simulink model "RobotX_ss_acoustics_1019_bbox"  (R2014a)
settings: Solver=FixedStepDiscrete  StartTime=0.0  StopTime=inf  FixedStep=.25  RelTol=1e-3
undefined symbols (not defined in the file): Com1, Com2, Com3, Com4, DiscIntNeverNeededParam, standard
libraries: xpcseriallib x14, dspmtrx3 x3, slrtlib x3, simulink x2, speedgoatlib x1, speedgoatlib_IO102 x1
(part 2 of 3)

== matlab function RobotX_ss_acoustics_1019_bbox/Main FSM/Start//Speedgate/entrance/GPSMove ==
  data: GoalNED input; X input; Finished output; valid output; Y input; Psi input; pts output
function [Finished,valid,pts] = GPSmove(GoalNED,X,Y,Psi)
%Written by Dylan DeGaetano on September 1, 2014
%Last edited by: Anderson Lebbad
%
%This function will go to a given NED cooridnate, last edit changed the
%goal pt and variable names

persistent Sample
if isempty(Sample)
Sample = 0;
end
Finished = 0;
pts = zeros(8,2);
%$Distance to object in meters
if Sample == 100
    Sample = 0;
end

if Sample == 0
    pts(1,1) = X+5*cos(Psi*pi/180);
    pts(1,2) = Y+5*cos(Psi*pi/180);
    pts(8,1) = GoalNED(1,1);
    pts(8,2) = GoalNED(1,2);
    pts(2,:) = pts(1,:) +(1*(GoalNED-pts(1,:))/7);
    pts(3,:) = pts(1,:) +(2*(GoalNED-pts(1,:))/7);
    pts(4,:) = pts(1,:) +(3*(GoalNED-pts(1,:))/7);
    pts(5,:) = pts(1,:) +(4*(GoalNED-pts(1,:))/7);
    pts(6,:) = pts(1,:) +(5*(GoalNED-pts(1,:))/7);
    pts(7,:) = pts(1,:) +(6*(GoalNED-pts(1,:))/7);
    Sample = 1; 
    valid = 1;
    
else 
    range = sqrt(sum((GoalNED - [X Y]).^2));
    if range <= 8
        Finished = 1;
    end
    valid = 0;
    Sample = Sample + 1;
end

== matlab function RobotX_ss_acoustics_1019_bbox/Main FSM/Start//Speedgate/exit/CalcTimes ==
  data: pts input; u input; Data output
function Data = calcTimes(pts, u)
%Written by Anderson Lebbad on August 9, 2014
%Last Edited: Dylan DeGaetano September 1, 2014

%Calculates times for the boat to get to points for a trajectory, and
%formats Data for communication

%Initialize
Data = zeros(24,1);
traj = zeros(8,3);
traj(:,1:2) = pts;



for k = 2:8
    %Calculate distance to travel from last point
    distTravel = sqrt(sum((pts(k-1,:)-pts(k,:)).^2));
    %Assume 1m per second speed
    traj(k,3) = traj(k-1,3) + distTravel;
    %Add time based off initial velocity to get to first point past initial
    if k == 2
        traj(k,3) = traj(k,3) + 2.5*abs(2-u);
    end
end


%Output Data
for i=1:8
    for j = 1:3
        Data(3*(i-1)+j) = traj(i,j);
    end
end

== matlab function RobotX_ss_acoustics_1019_bbox/Main FSM/Start//Speedgate/exit/GPSMove ==
  data: GoalNED input; X input; Finished output; valid output; Y input; Psi input; pts output
function [Finished,valid,pts] = GPSmove(GoalNED,X,Y,Psi)
%Written by Dylan DeGaetano on September 1, 2014
%Last edited by: Anderson Lebbad
%
%This function will go to a given NED cooridnate, last edit changed the
%goal pt and variable names

persistent Sample
if isempty(Sample)
Sample = 0;
end
Finished = 0;
pts = zeros(8,2);
%$Distance to object in meters
if Sample == 100
    Sample = 0;
end

if Sample == 0
    pts(1,1) = X+5*cos(Psi*pi/180);
    pts(1,2) = Y+5*cos(Psi*pi/180);
    pts(8,1) = GoalNED(1,1);
    pts(8,2) = GoalNED(1,2);
    pts(2,:) = pts(1,:) +(1*(GoalNED-pts(1,:))/7);
    pts(3,:) = pts(1,:) +(2*(GoalNED-pts(1,:))/7);
    pts(4,:) = pts(1,:) +(3*(GoalNED-pts(1,:))/7);
    pts(5,:) = pts(1,:) +(4*(GoalNED-pts(1,:))/7);
    pts(6,:) = pts(1,:) +(5*(GoalNED-pts(1,:))/7);
    pts(7,:) = pts(1,:) +(6*(GoalNED-pts(1,:))/7);
    Sample = 1; 
    valid = 1;
    
else 
    range = sqrt(sum((GoalNED - [X Y]).^2));
    if range <= 8
        Finished = 1;
    end
    valid = 0;
    Sample = Sample + 1;
end

== matlab function RobotX_ss_acoustics_1019_bbox/Main FSM/Termination/CalcTimes ==
  data: pts input; u input; Data output
function Data = calcTimes(pts, u)
%Written by Anderson Lebbad on August 9, 2014
%Last Edited: Dylan DeGaetano September 1, 2014

%Calculates times for the boat to get to points for a trajectory, and
%formats Data for communication

%Initialize
Data = zeros(24,1);
traj = zeros(8,3);
traj(:,1:2) = pts;



for k = 2:8
    %Calculate distance to travel from last point
    distTravel = sqrt(sum((pts(k-1,:)-pts(k,:)).^2));
    %Assume 1m per second speed
    traj(k,3) = traj(k-1,3) + distTravel;
    %Add time based off initial velocity to get to first point past initial
    if k == 2
        traj(k,3) = traj(k,3) + 2.5*abs(2-u);
    end
end


%Output Data
for i=1:8
    for j = 1:3
        Data(3*(i-1)+j) = traj(i,j);
    end
end

== matlab function RobotX_ss_acoustics_1019_bbox/Main FSM/Termination/GPSMove ==
  data: GoalNED input; X input; valid output; Y input; Psi input; pts output
function [valid,pts] = GPSmove(GoalNED,X,Y,Psi)
%Written by Dylan DeGaetano on September 1, 2014
%Last edited by: Anderson Lebbad
%
%This function will go to a given NED cooridnate, last edit changed the
%goal pt and variable names

persistent Sample
if isempty(Sample)
Sample = 0;
end

pts = zeros(8,2);
%$Distance to object in meters

if Sample == 0
    pts(1,1) = X+5*cos(Psi*pi/180);
    pts(1,2) = Y+5*cos(Psi*pi/180);
    pts(8,1) = GoalNED(1,1);
    pts(8,2) = GoalNED(1,2);
    pts(2,:) = pts(1,:) +(1*(GoalNED-pts(1,:))/7);
    pts(3,:) = pts(1,:) +(2*(GoalNED-pts(1,:))/7);
    pts(4,:) = pts(1,:) +(3*(GoalNED-pts(1,:))/7);
    pts(5,:) = pts(1,:) +(4*(GoalNED-pts(1,:))/7);
    pts(6,:) = pts(1,:) +(5*(GoalNED-pts(1,:))/7);
    pts(7,:) = pts(1,:) +(6*(GoalNED-pts(1,:))/7);
    Sample = 1; 
    valid = 1;
    
else
    valid = 0;
end

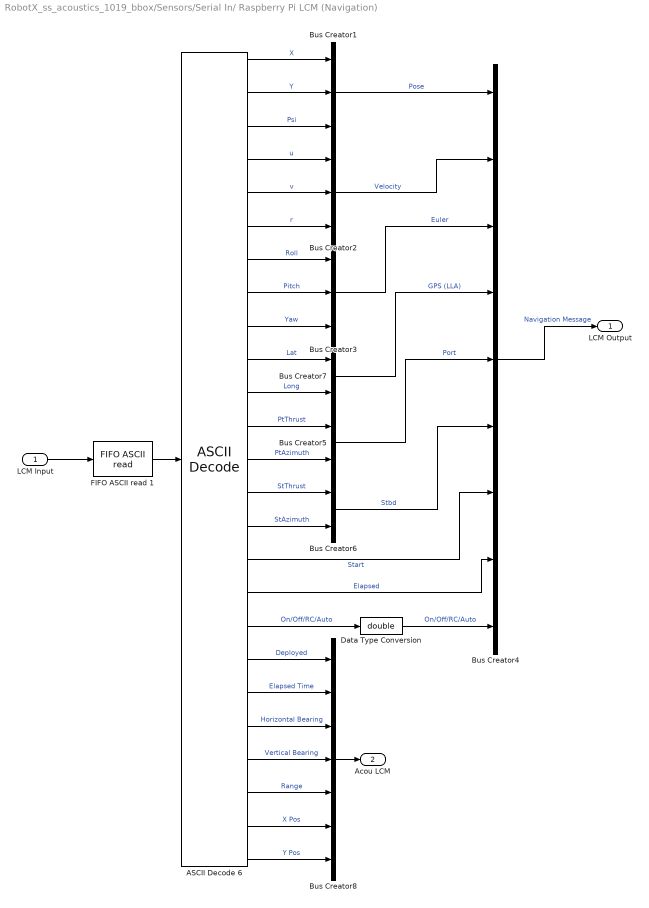
== system RobotX_ss_acoustics_1019_bbox/Sensors/Serial In/ Raspberry Pi LCM (Navigation) ==
  LCM Input : Inport
  ASCII Decode 6 : xpcseriallib/ASCII Decode   format=P1:%f P2:%f P3:%f V1:%f V2:%f V3:%f E1:%f E2:%f E3:%f Lat:%f Long:%f Pt1:%f Pt2:%f St1:%f St2:%f Start:%f Elapsed:%f RC:%d Deploy:%u Elapsed:%f Bearing1:%f Bearing2:%f Range:%f X_Pos:%f Y_Pos:%f \r\n  nvars=25  vartypes={}
  Bus Creator1 : BusCreator  Inputs=3
  Bus Creator2 : BusCreator  Inputs=3
  Bus Creator3 : BusCreator  Inputs=3
  Bus Creator4 : BusCreator  Inputs=9
  Bus Creator5 : BusCreator  Inputs=2
  Bus Creator6 : BusCreator  Inputs=2
  Bus Creator7 : BusCreator  Inputs=2
  Bus Creator8 : BusCreator  Inputs=7
  Data Type Conversion : DataTypeConversion  OutDataTypeStr=double
  FIFO ASCII read 1 : xpcseriallib/FIFO ASCII read   header={'P1:'}  term=[13 10]  hold=Zero output if no new data  enable=off  maxsize=1024  outputtype=8 bit uint null terminated  sampletime=-1
  LCM Output : Outport
  Acou LCM : Outport  Port=2
  wires:
  LCM Input/1 -> FIFO ASCII read 1/1
  FIFO ASCII read 1/1 -> ASCII Decode 6/1
  Bus Creator4/1 -> LCM Output/1  "Navigation Message"
  ASCII Decode 6/1 -> Bus Creator1/1  "X"
  ASCII Decode 6/2 -> Bus Creator1/2  "Y"
  ASCII Decode 6/3 -> Bus Creator1/3  "Psi"
  Bus Creator1/1 -> Bus Creator4/1  "Pose"
  ASCII Decode 6/4 -> Bus Creator2/1  "u"
  ASCII Decode 6/5 -> Bus Creator2/2  "v"
  Bus Creator2/1 -> Bus Creator4/2  "Velocity"
  ASCII Decode 6/7 -> Bus Creator3/1  "Roll"
  ASCII Decode 6/8 -> Bus Creator3/2  "Pitch"
  ASCII Decode 6/9 -> Bus Creator3/3  "Yaw"
  Bus Creator3/1 -> Bus Creator4/3  "Euler"
  Bus Creator5/1 -> Bus Creator4/5  "Port"
  Bus Creator6/1 -> Bus Creator4/6  "Stbd"
  ASCII Decode 6/14 -> Bus Creator6/1  "StThrust"
  ASCII Decode 6/15 -> Bus Creator6/2  "StAzimuth"
  ASCII Decode 6/12 -> Bus Creator5/1  "PtThrust"
  ASCII Decode 6/13 -> Bus Creator5/2  "PtAzimuth"
  ASCII Decode 6/16 -> Bus Creator4/7  "Start"
  ASCII Decode 6/17 -> Bus Creator4/8  "Elapsed"
  ASCII Decode 6/18 -> Data Type Conversion/1  "On/Off/RC/Auto"
  Data Type Conversion/1 -> Bus Creator4/9  "On/Off/RC/Auto"
  ASCII Decode 6/6 -> Bus Creator2/3  "r"
  ASCII Decode 6/10 -> Bus Creator7/1  "Lat"
  ASCII Decode 6/11 -> Bus Creator7/2  "Long"
  Bus Creator7/1 -> Bus Creator4/4  "GPS (LLA)"
  ASCII Decode 6/19 -> Bus Creator8/1  "Deployed"
  ASCII Decode 6/20 -> Bus Creator8/2  "Elapsed Time"
  ASCII Decode 6/21 -> Bus Creator8/3  "Horizontal Bearing"
  ASCII Decode 6/22 -> Bus Creator8/4  "Vertical Bearing"
  ASCII Decode 6/23 -> Bus Creator8/5  "Range"
  ASCII Decode 6/24 -> Bus Creator8/6  "X Pos"
  ASCII Decode 6/25 -> Bus Creator8/7  "Y Pos"
  Bus Creator8/1 -> Acou LCM/1

== system RobotX_ss_acoustics_1019_bbox/Sensors/Serial In/Acoustic LCM ==
  LCM Input : Inport
  Bus Creator : BusCreator  Inputs=2
  Bus Creator1 : BusCreator
  Bus Creator2 : BusCreator  Inputs=3
  Bus Selector : BusSelector  OutputSignals=Deployed,Elapsed Time,Horizontal Bearing,Vertical Bearing,Range,X Pos,Y Pos
  LCM Output : Outport
  wires:
  Bus Selector/3 -> Bus Creator/1  "<Horizontal Bearing>"
  Bus Selector/4 -> Bus Creator/2  "<Vertical Bearing>"
  Bus Creator/1 -> Bus Creator1/3  "Bearings"
  Bus Selector/2 -> Bus Creator1/2  "<Elapsed Time>"
  Bus Selector/1 -> Bus Creator1/1  "<Deployed>"
  Bus Creator1/1 -> LCM Output/1  "Acoustic Message"
  LCM Input/1 -> Bus Selector/1
  Bus Selector/5 -> Bus Creator2/1  "<Range>"
  Bus Selector/6 -> Bus Creator2/2  "<X Pos>"
  Bus Selector/7 -> Bus Creator2/3  "<Y Pos>"
  Bus Creator2/1 -> Bus Creator1/4  "Pose Estimate"

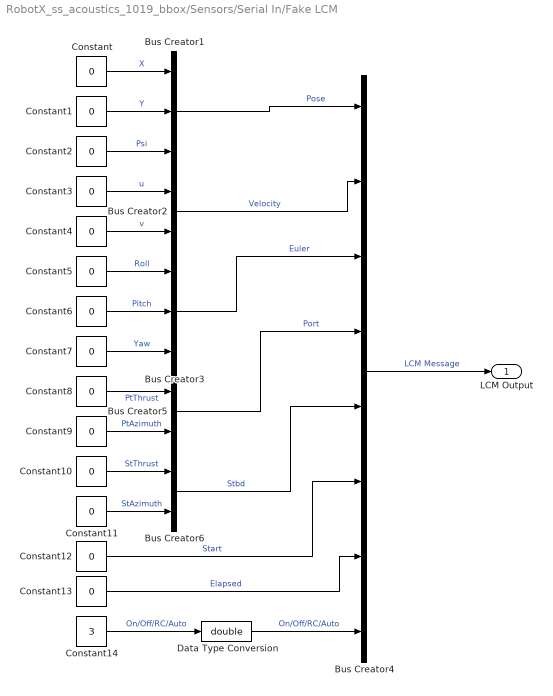
== system RobotX_ss_acoustics_1019_bbox/Sensors/Serial In/Fake LCM ==
  Bus Creator1 : BusCreator  Inputs=3
  Bus Creator2 : BusCreator  Inputs=2
  Bus Creator3 : BusCreator  Inputs=3
  Bus Creator4 : BusCreator  Inputs=8
  Bus Creator5 : BusCreator  Inputs=2
  Bus Creator6 : BusCreator  Inputs=2
  Constant{,1..13} (14 alike) : Constant  Value=0
  Constant14 : Constant  Value=3
  Data Type Conversion : DataTypeConversion  OutDataTypeStr=double
  LCM Output : Outport
  wires:
  Bus Creator4/1 -> LCM Output/1  "LCM Message"
  Constant/1 -> Bus Creator1/1  "X"
  Constant1/1 -> Bus Creator1/2  "Y"
  Constant2/1 -> Bus Creator1/3  "Psi"
  Bus Creator1/1 -> Bus Creator4/1  "Pose"
  Constant3/1 -> Bus Creator2/1  "u"
  Constant4/1 -> Bus Creator2/2  "v"
  Bus Creator2/1 -> Bus Creator4/2  "Velocity"
  Constant5/1 -> Bus Creator3/1  "Roll"
  Constant6/1 -> Bus Creator3/2  "Pitch"
  Constant7/1 -> Bus Creator3/3  "Yaw"
  Bus Creator3/1 -> Bus Creator4/3  "Euler"
  Bus Creator5/1 -> Bus Creator4/4  "Port"
  Bus Creator6/1 -> Bus Creator4/5  "Stbd"
  Constant10/1 -> Bus Creator6/1  "StThrust"
  Constant11/1 -> Bus Creator6/2  "StAzimuth"
  Constant8/1 -> Bus Creator5/1  "PtThrust"
  Constant9/1 -> Bus Creator5/2  "PtAzimuth"
  Constant12/1 -> Bus Creator4/6  "Start"
  Constant13/1 -> Bus Creator4/7  "Elapsed"
  Constant14/1 -> Data Type Conversion/1  "On/Off/RC/Auto"
  Data Type Conversion/1 -> Bus Creator4/8  "On/Off/RC/Auto"

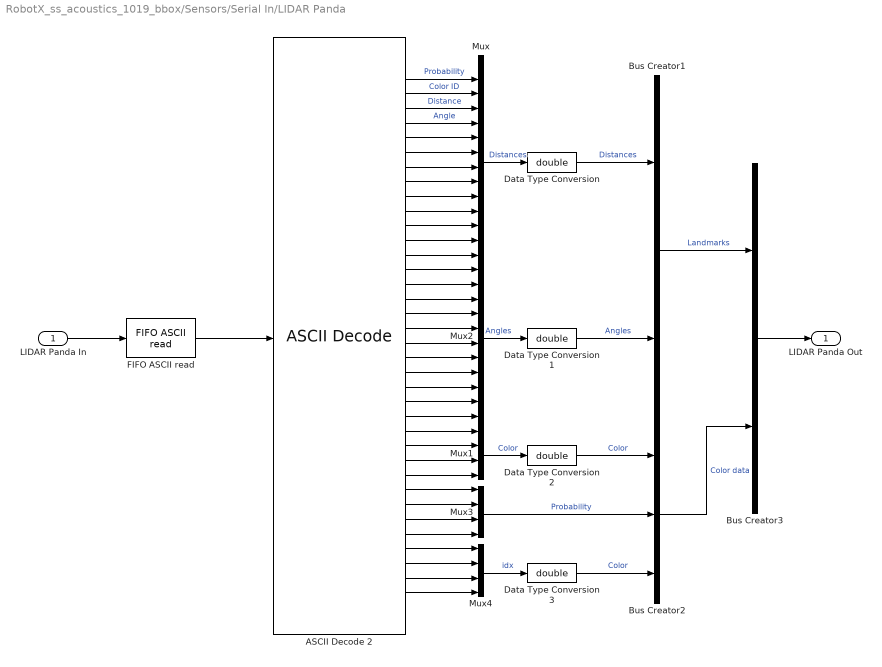
== system RobotX_ss_acoustics_1019_bbox/Sensors/Serial In/LIDAR Panda ==
  LIDAR Panda In : Inport
  ASCII Decode 2 : xpcseriallib/ASCII Decode   format=A:%d B:%d C:%d E:%d F:%d G:%d H:%d I:%d J:%d K:%d L:%d M:%d N:%d O:%d P:%d Q:%d R:%d S:%d T:%d U:%d V:%d W:%d X:%d C1:%d C2:%d C3:%d C4:%d P1:%f P2:%f P3:%f P4:%f I1:%d I2:%d I3:%d I4:%d \r\n  nvars=36  vartypes={}
  Bus Creator1 : BusCreator  Inputs=2
  Bus Creator2 : BusCreator  Inputs=3
  Bus Creator3 : BusCreator  Inputs=2
  Data Type Conversion{,1..3} (4 alike) : DataTypeConversion  OutDataTypeStr=double
  "FIFO ASCII read " : xpcseriallib/FIFO ASCII read   header={'A:'}  term=[13 10]  hold=Zero output if no new data  enable=off  maxsize=1024  outputtype=8 bit uint null terminated  sampletime=-1
  Mux : Mux  Inputs=12
  Mux1 : Mux
  Mux2 : Mux  Inputs=12
  Mux3 : Mux
  Mux4 : Mux
  LIDAR Panda Out : Outport
  wires:
  LIDAR Panda In/1 -> "FIFO ASCII read "/1
  "FIFO ASCII read "/1 -> ASCII Decode 2/1
  ASCII Decode 2/3 -> Mux/3  "Distance"
  ASCII Decode 2/2 -> Mux/2  "Color ID"
  ASCII Decode 2/4 -> Mux/4  "Angle"
  ASCII Decode 2/1 -> Mux/1  "Probability"
  ASCII Decode 2/7 -> Mux/7
  ASCII Decode 2/10 -> Mux/10
  ASCII Decode 2/11 -> Mux/11
  ASCII Decode 2/6 -> Mux/6
  ASCII Decode 2/8 -> Mux/8
  ASCII Decode 2/9 -> Mux/9
  ASCII Decode 2/12 -> Mux/12
  ASCII Decode 2/5 -> Mux/5
  ASCII Decode 2/13 -> Mux2/1
  ASCII Decode 2/15 -> Mux2/3
  ASCII Decode 2/22 -> Mux2/10
  ASCII Decode 2/23 -> Mux2/11
  ASCII Decode 2/17 -> Mux2/5
  ASCII Decode 2/18 -> Mux2/6
  ASCII Decode 2/14 -> Mux2/2
  ASCII Decode 2/24 -> Mux2/12
  ASCII Decode 2/20 -> Mux2/8
  ASCII Decode 2/19 -> Mux2/7
  ASCII Decode 2/21 -> Mux2/9
  ASCII Decode 2/16 -> Mux2/4
  ASCII Decode 2/25 -> Mux1/1
  ASCII Decode 2/28 -> Mux1/4
  ASCII Decode 2/26 -> Mux1/2
  ASCII Decode 2/27 -> Mux1/3
  ASCII Decode 2/30 -> Mux3/2
  ASCII Decode 2/31 -> Mux3/3
  ASCII Decode 2/32 -> Mux3/4
  ASCII Decode 2/29 -> Mux3/1
  ASCII Decode 2/36 -> Mux4/4
  ASCII Decode 2/34 -> Mux4/2
  ASCII Decode 2/35 -> Mux4/3
  ASCII Decode 2/33 -> Mux4/1
  Mux/1 -> Data Type Conversion/1  "Distances"
  Mux2/1 -> Data Type Conversion1/1  "Angles"
  Mux1/1 -> Data Type Conversion2/1  "Color"
  Mux3/1 -> Bus Creator2/2  "Probability"
  Mux4/1 -> Data Type Conversion3/1  "idx"
  Bus Creator1/1 -> Bus Creator3/1  "Landmarks"
  Bus Creator2/1 -> Bus Creator3/2  "Color data"
  Bus Creator3/1 -> LIDAR Panda Out/1
  Data Type Conversion/1 -> Bus Creator1/1  "Distances"
  Data Type Conversion1/1 -> Bus Creator1/2  "Angles"
  Data Type Conversion2/1 -> Bus Creator2/1  "Color"
  Data Type Conversion3/1 -> Bus Creator2/3  "Color"

== system RobotX_ss_acoustics_1019_bbox/Sensors/Serial In/Subsystem ==
  Bus Creator : BusCreator  Inputs=3
  Bus Creator1 : BusCreator  Inputs=2
  Bus Creator2 : BusCreator  Inputs=2
  Constant : Constant  Value=zeros(12,1)
  Constant1 : Constant  Value=zeros(12,1)
  Constant2 : Constant  Value=zeros(4,1)
  Constant3 : Constant  Value=zeros(4,1)
  Constant4 : Constant  Value=zeros(4,1)
  Fake Panda : Outport
  wires:
  Constant/1 -> Bus Creator1/1  "Distances"
  Constant1/1 -> Bus Creator1/2  "Angles"
  Constant2/1 -> Bus Creator/1  "Color"
  Constant3/1 -> Bus Creator/2  "Probability"
  Constant4/1 -> Bus Creator/3  "idx"
  Bus Creator1/1 -> Bus Creator2/1  "Landmarks"
  Bus Creator/1 -> Bus Creator2/2  "Color data"
  Bus Creator2/1 -> Fake Panda/1  "Lidar Data Input"

== system RobotX_ss_acoustics_1019_bbox/Sensors/Serial In/data log ==
  Sensors signal : Inport
  Bus Selector3 : BusSelector  OutputSignals=Navigation Message,Lidar Data Input,Acoustic Message
  Bus to Vector : BusToVector
  Bus to Vector1 : BusToVector
  Bus to Vector2 : BusToVector
  Scope 1 : slrtlib/Displays and Logging/Scope   scopeno=4  scopetype=File  autostart=on  viewmode=Graphical redraw  formatstr='%15.6f'  grid=on  ylimits=[0,0]  nosamples=28800  noprepostsamples=0  interleave=1  triggermode=FreeRun  triggersignal=1  trigsignalfromport=off  triggerlevel=0.0  triggerslope=Either  triggerscope=1  triggersample=0  filename=LM1_<%%%>.dat  mode=Lazy  writesize=512  autorestart=on  dynamicfilemode=on  maxwritefilesize=512*1024^2
  Scope 2 : slrtlib/Displays and Logging/Scope   scopeno=1  scopetype=File  autostart=on  viewmode=Graphical redraw  formatstr='%15.6f'  grid=on  ylimits=[0,0]  nosamples=28800  noprepostsamples=0  interleave=1  triggermode=FreeRun  triggersignal=1  trigsignalfromport=off  triggerlevel=0.0  triggerslope=Either  triggerscope=1  triggersample=0  filename=NAV1_<%%%>.dat  mode=Lazy  writesize=512  autorestart=on  dynamicfilemode=on  maxwritefilesize=512*1024^2
  Scope 3 : slrtlib/Displays and Logging/Scope   scopeno=2  scopetype=File  autostart=on  viewmode=Graphical redraw  formatstr='%15.6f'  grid=on  ylimits=[0,0]  nosamples=28800  noprepostsamples=0  interleave=1  triggermode=FreeRun  triggersignal=1  trigsignalfromport=off  triggerlevel=0.0  triggerslope=Either  triggerscope=1  triggersample=0  filename=ACO1_<%%%>.dat  mode=Lazy  writesize=512  autorestart=on  dynamicfilemode=on  maxwritefilesize=512*1024^2
  wires:
  Sensors signal/1 -> Bus Selector3/1
  Bus to Vector/1 -> Scope 2/1
  Bus Selector3/1 -> Bus to Vector/1  "<Navigation Message>"
  Bus to Vector1/1 -> Scope 1/1
  Bus to Vector2/1 -> Scope 3/1
  Bus Selector3/3 -> Bus to Vector2/1  "<Acoustic Message>"
  Bus Selector3/2 -> Bus to Vector1/1  "<Lidar Data Input>"

== system RobotX_ss_acoustics_1019_bbox/Main FSM/Acoustic FSM/Acoustics Pt1/Output Heirarchy ==
  Data : Inport
  Sensors : Inport  Port=2
  Acoustic Active : Constant
  Bus Creator2 : BusCreator  Inputs=3
  Bus Creator3 : BusCreator  Inputs=3
  Bus Creator5 : BusCreator  Inputs=2
  Constant : Constant
  Constant3 : Constant
  Lidar Mode : Constant
  Outputs : Outport
  wires:
  Sensors/1 -> Bus Creator5/2  "Sensors"
  Bus Creator5/1 -> Outputs/1  "Output Signals"
  Constant/1 -> Bus Creator2/1  "Valid"
  Constant3/1 -> Bus Creator2/2  "Control Mode"
  Data/1 -> Bus Creator2/3  "Data"
  Bus Creator2/1 -> Bus Creator3/1  "Navigation Outputs"
  Acoustic Active/1 -> Bus Creator3/2  "Acoustic Active"
  Lidar Mode/1 -> Bus Creator3/3  "Lidar Mode"
  Bus Creator3/1 -> Bus Creator5/1  "Outputs"

== system RobotX_ss_acoustics_1019_bbox/Main FSM/Acoustic FSM/Acoustics Pt2/Output Heirarchy ==
  Data : Inport
  Sensors : Inport  Port=2
  Acoustic Active : Constant
  Bus Creator2 : BusCreator  Inputs=3
  Bus Creator3 : BusCreator  Inputs=3
  Bus Creator5 : BusCreator  Inputs=2
  Constant : Constant
  Constant3 : Constant
  Lidar Mode : Constant
  Outputs : Outport
  wires:
  Sensors/1 -> Bus Creator5/2  "Sensors"
  Bus Creator5/1 -> Outputs/1  "Output Signals"
  Constant/1 -> Bus Creator2/1  "Valid"
  Constant3/1 -> Bus Creator2/2  "Control Mode"
  Data/1 -> Bus Creator2/3  "Data"
  Bus Creator2/1 -> Bus Creator3/1  "Navigation Outputs"
  Acoustic Active/1 -> Bus Creator3/2  "Acoustic Active"
  Lidar Mode/1 -> Bus Creator3/3  "Lidar Mode"
  Bus Creator3/1 -> Bus Creator5/1  "Outputs"

== system RobotX_ss_acoustics_1019_bbox/Main FSM/Acoustic FSM/Acoustics Pt3/Output Heirarchy ==
  Data : Inport
  Sensors : Inport  Port=2
  Acoustic Active : Constant
  Bus Creator2 : BusCreator  Inputs=3
  Bus Creator3 : BusCreator  Inputs=3
  Bus Creator5 : BusCreator  Inputs=2
  Constant : Constant
  Constant3 : Constant
  Lidar Mode : Constant
  Outputs : Outport
  wires:
  Sensors/1 -> Bus Creator5/2  "Sensors"
  Bus Creator5/1 -> Outputs/1  "Output Signals"
  Constant/1 -> Bus Creator2/1  "Valid"
  Constant3/1 -> Bus Creator2/2  "Control Mode"
  Data/1 -> Bus Creator2/3  "Data"
  Bus Creator2/1 -> Bus Creator3/1  "Navigation Outputs"
  Acoustic Active/1 -> Bus Creator3/2  "Acoustic Active"
  Lidar Mode/1 -> Bus Creator3/3  "Lidar Mode"
  Bus Creator3/1 -> Bus Creator5/1  "Outputs"

== system RobotX_ss_acoustics_1019_bbox/Main FSM/Acoustic FSM/Move 1/Output Reassign ==
  Vaild : Inport
  Data : Inport  Port=2
  Sensors : Inport  Port=3
  Acoustic Active : Constant  Value=0
  Bus Creator2 : BusCreator  Inputs=3
  Bus Creator3 : BusCreator  Inputs=3
  Bus Creator5 : BusCreator  Inputs=2
  Constant3 : Constant  Value=0
  Lidar Mode : Constant  Value=0
  Outputs : Outport
  wires:
  Sensors/1 -> Bus Creator5/2  "Sensors"
  Bus Creator5/1 -> Outputs/1  "Output Signals"
  Vaild/1 -> Bus Creator2/1  "Valid"
  Constant3/1 -> Bus Creator2/2  "Control Mode"
  Data/1 -> Bus Creator2/3  "Data"
  Bus Creator2/1 -> Bus Creator3/1  "Navigation Outputs"
  Acoustic Active/1 -> Bus Creator3/2  "Acoustic Active"
  Lidar Mode/1 -> Bus Creator3/3  "Lidar Mode"
  Bus Creator3/1 -> Bus Creator5/1  "Outputs"

== system RobotX_ss_acoustics_1019_bbox/Main FSM/Acoustic FSM/Move 2/Output Reassign ==
  Vaild : Inport
  Data : Inport  Port=2
  Sensors : Inport  Port=3
  Acoustic Active : Constant  Value=0
  Bus Creator2 : BusCreator  Inputs=3
  Bus Creator3 : BusCreator  Inputs=3
  Bus Creator5 : BusCreator  Inputs=2
  Constant3 : Constant  Value=0
  Lidar Mode : Constant  Value=0
  Outputs : Outport
  wires:
  Sensors/1 -> Bus Creator5/2  "Sensors"
  Bus Creator5/1 -> Outputs/1  "Output Signals"
  Vaild/1 -> Bus Creator2/1  "Valid"
  Constant3/1 -> Bus Creator2/2  "Control Mode"
  Data/1 -> Bus Creator2/3  "Data"
  Bus Creator2/1 -> Bus Creator3/1  "Navigation Outputs"
  Acoustic Active/1 -> Bus Creator3/2  "Acoustic Active"
  Lidar Mode/1 -> Bus Creator3/3  "Lidar Mode"
  Bus Creator3/1 -> Bus Creator5/1  "Outputs"

== system RobotX_ss_acoustics_1019_bbox/Main FSM/Acoustic FSM/Move 3/Output Reassign ==
  Vaild : Inport
  Data : Inport  Port=2
  Sensors : Inport  Port=3
  Acoustic Active : Constant  Value=0
  Bus Creator2 : BusCreator  Inputs=3
  Bus Creator3 : BusCreator  Inputs=3
  Bus Creator5 : BusCreator  Inputs=2
  Constant3 : Constant  Value=0
  Lidar Mode : Constant  Value=0
  Outputs : Outport
  wires:
  Sensors/1 -> Bus Creator5/2  "Sensors"
  Bus Creator5/1 -> Outputs/1  "Output Signals"
  Vaild/1 -> Bus Creator2/1  "Valid"
  Constant3/1 -> Bus Creator2/2  "Control Mode"
  Data/1 -> Bus Creator2/3  "Data"
  Bus Creator2/1 -> Bus Creator3/1  "Navigation Outputs"
  Acoustic Active/1 -> Bus Creator3/2  "Acoustic Active"
  Lidar Mode/1 -> Bus Creator3/3  "Lidar Mode"
  Bus Creator3/1 -> Bus Creator5/1  "Outputs"

== system RobotX_ss_acoustics_1019_bbox/Main FSM/Acoustic FSM/Point/Output Heirarchy ==
  Data : Inport
  Sensors : Inport  Port=2
  Acoustic Active : Constant
  Bus Creator2 : BusCreator  Inputs=3
  Bus Creator3 : BusCreator  Inputs=3
  Bus Creator5 : BusCreator  Inputs=2
  Constant : Constant
  Constant3 : Constant
  Lidar Mode : Constant
  Outputs : Outport
  wires:
  Sensors/1 -> Bus Creator5/2  "Sensors"
  Bus Creator5/1 -> Outputs/1  "Output Signals"
  Constant/1 -> Bus Creator2/1  "Valid"
  Constant3/1 -> Bus Creator2/2  "Control Mode"
  Data/1 -> Bus Creator2/3  "Data"
  Bus Creator2/1 -> Bus Creator3/1  "Navigation Outputs"
  Acoustic Active/1 -> Bus Creator3/2  "Acoustic Active"
  Lidar Mode/1 -> Bus Creator3/3  "Lidar Mode"
  Bus Creator3/1 -> Bus Creator5/1  "Outputs"

== system RobotX_ss_acoustics_1019_bbox/Main FSM/Start//Speedgate/GPS Move/Output Reassign ==
  Vaild : Inport
  Data : Inport  Port=2
  Sensors : Inport  Port=3
  Acoustic Active : Constant  Value=0
  Bus Creator2 : BusCreator  Inputs=3
  Bus Creator3 : BusCreator  Inputs=3
  Bus Creator5 : BusCreator  Inputs=2
  Constant3 : Constant  Value=0
  Lidar Mode : Constant  Value=0
  Outputs : Outport
  wires:
  Sensors/1 -> Bus Creator5/2  "Sensors"
  Bus Creator5/1 -> Outputs/1  "Output Signals"
  Vaild/1 -> Bus Creator2/1  "Valid"
  Constant3/1 -> Bus Creator2/2  "Control Mode"
  Data/1 -> Bus Creator2/3  "Data"
  Bus Creator2/1 -> Bus Creator3/1  "Navigation Outputs"
  Acoustic Active/1 -> Bus Creator3/2  "Acoustic Active"
  Lidar Mode/1 -> Bus Creator3/3  "Lidar Mode"
  Bus Creator3/1 -> Bus Creator5/1  "Outputs"

== system RobotX_ss_acoustics_1019_bbox/Main FSM/Start//Speedgate/entrance/Output Reassign ==
  Vaild : Inport
  Data : Inport  Port=2
  Sensors : Inport  Port=3
  Acoustic Active : Constant  Value=0
  Bus Creator2 : BusCreator  Inputs=3
  Bus Creator3 : BusCreator  Inputs=3
  Bus Creator5 : BusCreator  Inputs=2
  Constant3 : Constant  Value=0
  Lidar Mode : Constant  Value=0
  Outputs : Outport
  wires:
  Sensors/1 -> Bus Creator5/2  "Sensors"
  Bus Creator5/1 -> Outputs/1  "Output Signals"
  Vaild/1 -> Bus Creator2/1  "Valid"
  Constant3/1 -> Bus Creator2/2  "Control Mode"
  Data/1 -> Bus Creator2/3  "Data"
  Bus Creator2/1 -> Bus Creator3/1  "Navigation Outputs"
  Acoustic Active/1 -> Bus Creator3/2  "Acoustic Active"
  Lidar Mode/1 -> Bus Creator3/3  "Lidar Mode"
  Bus Creator3/1 -> Bus Creator5/1  "Outputs"

== system RobotX_ss_acoustics_1019_bbox/Main FSM/Start//Speedgate/exit/Output Reassign ==
  Vaild : Inport
  Data : Inport  Port=2
  Sensors : Inport  Port=3
  Acoustic Active : Constant  Value=0
  Bus Creator2 : BusCreator  Inputs=3
  Bus Creator3 : BusCreator  Inputs=3
  Bus Creator5 : BusCreator  Inputs=2
  Constant3 : Constant  Value=0
  Lidar Mode : Constant  Value=0
  Outputs : Outport
  wires:
  Sensors/1 -> Bus Creator5/2  "Sensors"
  Bus Creator5/1 -> Outputs/1  "Output Signals"
  Vaild/1 -> Bus Creator2/1  "Valid"
  Constant3/1 -> Bus Creator2/2  "Control Mode"
  Data/1 -> Bus Creator2/3  "Data"
  Bus Creator2/1 -> Bus Creator3/1  "Navigation Outputs"
  Acoustic Active/1 -> Bus Creator3/2  "Acoustic Active"
  Lidar Mode/1 -> Bus Creator3/3  "Lidar Mode"
  Bus Creator3/1 -> Bus Creator5/1  "Outputs"

== matlab function RobotX_ss_acoustics_1019_bbox/Main FSM/Termination/LLA to NED ==
  data: GoalLLA input; GoalNED output; NED_origin input
function GoalNED = LLA2NEDfun(GoalLLA,NED_origin)
%Written by Anderson Lebbad on September 20, 2014
%Last edited by:
%
%This function converts a target Latitude, Longitude, Altitude (LLA) point
%into North, East, Down (NED) coordinates

%First convert to earth centered, earth fixed frame
GoalECEF = lla2ecef([GoalLLA*(pi/180), 0]');
%Then convert from ECEF to North East Down
GoalNEDvect = ecef2ned(NED_origin'*(pi/180),GoalECEF);
GoalNED = GoalNEDvect(1:2)';

end

function x_ecef = lla2ecef(x_lla)
% LLE2ECEF: Converts from geodetic latitude, longitude, and altitude to earth-centered earth-fixed Cartesian coordinates
% INPUT: latitude phi (rad), longitude lambda (rad), altitude h (m)
% OUTPUT: [x, y, z]' (m) earth-centered earth-fixed Cartesian coordinates
    a = 6378137; % equatorial radius of ellipsoid (semi-major axis) (m)
    b = 6356752; % polar axis radius of ellipsoid (semi-minor axis) (m)

    phi = x_lla(1);
    lambda = x_lla(2);
    h = x_lla(3);
    
    % auxiliar quantities f, e, and N
    f = (a-b)/a;
    e = f*(2-f);
    N = a/sqrt(1-(e*sin(phi))^2);
    x_ecef = [(N+h)*cos(phi)*cos(lambda); (N+h)*cos(phi)*sin(lambda); (N*(1-e^2)+h)*sin(phi)];
end

function [x_ned] = ecef2ned(ned_lla, x_ecef)
% ECEF2NED Converts from earth-centered, earth-fixed Cartesian coordinates to tangent plane
% INPUT:
% 1) x_ecef=[x,y,z]' (m) earth-centered, earth-fixed Cartesian coordinates
% 2) ned_lla=[phi,lambda]' consiting of latitude phi (rad), longitude lambda (rad) of NED origin
% OUTPUT:
% 1) x_ned=[x,y,z]' (m) in NED coordinate system with the origin [phi,lambda]'

    phi = ned_lla(1);
    lambda = ned_lla(2);

    % transformation  matrix
    T = [-sin(phi)*cos(lambda) -sin(phi)*sin(lambda)  cos(phi)
         -sin(lambda)           cos(lambda)           0
          cos(phi)*cos(lambda)   cos(phi)*sin(lambda)  sin(phi)];

     x_ned = T*(x_ecef-lla2ecef([phi, lambda, 0]')); % convert to NED
     x_ned(3) = -x_ned(3);
end

== matlab function RobotX_ss_acoustics_1019_bbox/Main FSM/Acoustic FSM/Acoustics Pt1/Ping Point ==
  data: acousticPose output; Deployed input; Finished output; X input; Y input; Psi input; HorizBearing input; ElapsedTime input; Data output
function [acousticPose,Finished,Data] = PingPoint(Deployed,X,Y,Psi,...
    HorizBearing,ElapsedTime)
%Written by Anderson Lebbad on September 12, 2014
%Last Edited: September 14 - waits for boom deployment

%This function causes the vessel to spin in place until a ping is detected,
%then orients itself towards the direction of the source of that ping

persistent holdPose Pinged aveHeading First aveXY

if isempty(holdPose)
    holdPose = [X Y Psi];
    Pinged = 0;
    aveHeading = [0 0];
    aveXY = [0 0];
    First = 1;
end

%Initialize Data variable
Data = zeros(24,1);
Finished = 0;

%Angular offset (indirect rate control)
offset = 5;

%Wait for the boom to be lowered
if Deployed == 1
    %If the boat has not heard a ping yet, spin
    if Pinged == 0
        holdPose(3) = mod(Psi + offset,360);
    end
    
    %If the ping is less than 250 milliseconds (a timestep) then point at the
    %direction of sound
    if ElapsedTime < 250 && abs(HorizBearing) < 35
        if (abs(HorizBearing) >= 15 || First)
            holdPose(3) = mod(Psi + HorizBearing,360);
            Pinged = 1;
            First = 0;
        end
        aveHeading(1) = (aveHeading(1)*aveHeading(2)+Psi+HorizBearing)/(aveHeading(2)+1);
        aveHeading(2) = aveHeading(2)+1;
        aveXY(1) = (aveXY(1)*(aveHeading(2)-1)+X)/aveHeading(2);
        aveXY(2) = (aveXY(2)*(aveHeading(2)-1)+Y)/aveHeading(2);
    end
end

acousticPose = [aveXY aveHeading(1)];

if aveHeading(2) >= 16
    Finished = 1;
end

%Set desired pose
Data(1) = holdPose(1);
Data(2) = holdPose(2);
Data(3) = holdPose(3);

== matlab function RobotX_ss_acoustics_1019_bbox/Sensors/Serial In/Data Update2 ==
  data: Valid input; ControlMode input; V output; C output; L output; A output; Data input; D1 output; D2 output; D3 output; D4 output; D5 output; D6 output; D7 output; D8 output; D9 output; D10 output; D11 output; D12 output; D13 output; D14 output; D15 output; D16 output; D17 output; D18 output; D19 output; D20 output; D21 output; D22 output; D23 output; D24 output; Activate input
function [V,C,L,A,D1,D2,D3,D4,D5,D6,D7,D8,D9,D10,D11,D12,D13,D14,D15,D16,D17,...
    D18,D19,D20,D21,D22,D23,D24] = dataSplit(Valid,ControlMode,Data,Activate)
%Written by Anderson Lebbad on August 10, 2014
%Last Edited by: Anderson Lebbad on September 11, 2014

%This function splits the data vector into the twelve channels it is
%composed of for communication

persistent HoldData

if isempty(HoldData)
    HoldData = zeros(26,1);
    HoldData(2) = 2;
end

if Valid == 1
    HoldData(1) = Valid;
    HoldData(2) = ControlMode;
    HoldData(3) = Data(1);
    HoldData(4) = Data(2);
    HoldData(5) = Data(3);
    HoldData(6) = Data(4);
    HoldData(7) = Data(5);
    HoldData(8) = Data(6);
    HoldData(9) = Data(7);
    HoldData(10) = Data(8);
    HoldData(11) = Data(9);
    HoldData(12) = Data(10);
    HoldData(13) = Data(11);
    HoldData(14) = Data(12);
    HoldData(15) = Data(13);
    HoldData(16) = Data(14);
    HoldData(17) = Data(15);
    HoldData(18) = Data(16);
    HoldData(19) = Data(17);
    HoldData(20) = Data(18);
    HoldData(21) = Data(19);
    HoldData(22) = Data(20);
    HoldData(23) = Data(21);
    HoldData(24) = Data(22);
    HoldData(25) = Data(23);
    HoldData(26) = Data(24);
end

V = HoldData(1);
C = HoldData(2);
L = 8;
A = Activate;
D1 = HoldData(3);
D2 = HoldData(4);
D3 = HoldData(5);
D4 = HoldData(6);
D5 = HoldData(7);
D6 = HoldData(8);
D7 = HoldData(9);
D8 = HoldData(10);
D9 = HoldData(11);
D10 = HoldData(12);
D11 = HoldData(13);
D12 = HoldData(14);
D13 = HoldData(15);
D14 = HoldData(16);
D15 = HoldData(17);
D16 = HoldData(18);
D17 = HoldData(19);
D18 = HoldData(20);
D19 = HoldData(21);
D20 = HoldData(22);
D21 = HoldData(23);
D22 = HoldData(24);
D23 = HoldData(25);
D24 = HoldData(26);

end

== matlab function RobotX_ss_acoustics_1019_bbox/Main FSM/Acoustic FSM/Acoustics Pt2/Ping Point ==
  data: acousticPose output; Deployed input; Finished output; X input; Y input; Psi input; HorizBearing input; ElapsedTime input; Data output
function [acousticPose,Finished,Data] = PingPoint(Deployed,X,Y,Psi,...
    HorizBearing,ElapsedTime)
%Written by Anderson Lebbad on September 12, 2014
%Last Edited: September 14 - waits for boom deployment

%This function causes the vessel to spin in place until a ping is detected,
%then orients itself towards the direction of the source of that ping

persistent holdPose Pinged aveHeading First aveXY

if isempty(holdPose)
    holdPose = [X Y Psi];
    Pinged = 0;
    aveHeading = [0 0];
    aveXY = [0 0];
    First = 1;
end

%Initialize Data variable
Data = zeros(24,1);
Finished = 0;

%Angular offset (indirect rate control)
offset = 5;

%Wait for the boom to be lowered
if Deployed == 1
    %If the boat has not heard a ping yet, spin
    if Pinged == 0
        holdPose(3) = mod(Psi + offset,360);
    end
    
    %If the ping is less than 250 milliseconds (a timestep) then point at the
    %direction of sound
    if ElapsedTime < 250 && abs(HorizBearing) < 35
        if (abs(HorizBearing) >= 15 || First)
            holdPose(3) = mod(Psi + HorizBearing,360);
            Pinged = 1;
            First = 0;
        end
        aveHeading(1) = (aveHeading(1)*aveHeading(2)+Psi+HorizBearing)/(aveHeading(2)+1);
        aveHeading(2) = aveHeading(2)+1;
        aveXY(1) = (aveXY(1)*(aveHeading(2)-1)+X)/aveHeading(2);
        aveXY(2) = (aveXY(2)*(aveHeading(2)-1)+Y)/aveHeading(2);
    end
end

acousticPose = [aveXY aveHeading(1)];

if aveHeading(2) >= 16
    Finished = 1;
end

%Set desired pose
Data(1) = holdPose(1);
Data(2) = holdPose(2);
Data(3) = holdPose(3);

== matlab function RobotX_ss_acoustics_1019_bbox/Main FSM/Acoustic FSM/Move 2/CalcTimes ==
  data: pts input; u input; Data output
function Data = calcTimes(pts, u)
%Written by Anderson Lebbad on August 9, 2014
%Last Edited: Dylan DeGaetano September 1, 2014

%Calculates times for the boat to get to points for a trajectory, and
%formats Data for communication

%Initialize
Data = zeros(24,1);
traj = zeros(8,3);
traj(:,1:2) = pts;



for k = 2:8
    %Calculate distance to travel from last point
    distTravel = sqrt(sum((pts(k-1,:)-pts(k,:)).^2));
    %Assume 1m per second speed
    traj(k,3) = traj(k-1,3) + distTravel;
    %Add time based off initial velocity to get to first point past initial
    if k == 2
        traj(k,3) = traj(k,3) + 2.5*abs(2-u);
    end
end


%Output Data
for i=1:8
    for j = 1:3
        Data(3*(i-1)+j) = traj(i,j);
    end
end

== matlab function RobotX_ss_acoustics_1019_bbox/Main FSM/Start//Speedgate/GPS Move/CalcTimes ==
  data: pts input; u input; Data output
function Data = calcTimes(pts, u)
%Written by Anderson Lebbad on August 9, 2014
%Last Edited: Dylan DeGaetano September 1, 2014

%Calculates times for the boat to get to points for a trajectory, and
%formats Data for communication

%Initialize
Data = zeros(24,1);
traj = zeros(8,3);
traj(:,1:2) = pts;



for k = 2:8
    %Calculate distance to travel from last point
    distTravel = sqrt(sum((pts(k-1,:)-pts(k,:)).^2));
    %Assume 1m per second speed
    traj(k,3) = traj(k-1,3) + distTravel;
    %Add time based off initial velocity to get to first point past initial
    if k == 2
        traj(k,3) = traj(k,3) + 2.5*abs(2-u);
    end
end


%Output Data
for i=1:8
    for j = 1:3
        Data(3*(i-1)+j) = traj(i,j);
    end
end

== matlab function RobotX_ss_acoustics_1019_bbox/Main FSM/Start//Speedgate/GPS Move/GPSMove ==
  data: GoalNED input; X input; Finished output; valid output; Y input; Psi input; pts output
function [Finished,valid,pts] = GPSmove(GoalNED,X,Y,Psi)
%Written by Dylan DeGaetano on September 1, 2014
%Last edited by: Anderson Lebbad
%
%This function will go to a given NED cooridnate, last edit changed the
%goal pt and variable names

persistent Sample
if isempty(Sample)
Sample = 0;
end
Finished = 0;
pts = zeros(8,2);
%$Distance to object in meters
if Sample == 100
    Sample = 0;
end

if Sample == 0
    pts(1,1) = X+5*cos(Psi*pi/180);
    pts(1,2) = Y+5*cos(Psi*pi/180);
    pts(8,1) = GoalNED(1,1);
    pts(8,2) = GoalNED(1,2);
    pts(2,:) = pts(1,:) +(1*(GoalNED-pts(1,:))/7);
    pts(3,:) = pts(1,:) +(2*(GoalNED-pts(1,:))/7);
    pts(4,:) = pts(1,:) +(3*(GoalNED-pts(1,:))/7);
    pts(5,:) = pts(1,:) +(4*(GoalNED-pts(1,:))/7);
    pts(6,:) = pts(1,:) +(5*(GoalNED-pts(1,:))/7);
    pts(7,:) = pts(1,:) +(6*(GoalNED-pts(1,:))/7);
    Sample = 1; 
    valid = 1;
    
else 
    range = sqrt(sum((GoalNED - [X Y]).^2));
    if range <= 8
        Finished = 1;
    end
    valid = 0;
    Sample = Sample + 1;
end

== matlab function RobotX_ss_acoustics_1019_bbox/Main FSM/Start//Speedgate/Main Enabler ==
  data: taskSelector output; GpsEn output; aimEn output; deadEn output; ssgateTask input; GpsFin input; AimFin input
function [taskSelector,GpsEn,aimEn,deadEn]=Startgate_Enabler(ssgateTask,...
    GpsFin,AimFin)
%Written by Anderson Lebbad on July 19, 2013
%Last Edited: Dylan DeGaetano on September ,4 2014
%   Substring search for task was written in
%   Case switches were redundant, combined with first set of if statements

%Changes the value of MainMode and the enablers for the tasks within the
%Main FSM.

% Initialize enable signals
GpsEn = 0;
aimEn =0;
deadEn = 0;

% Convert main task indicator to a string
ssgateTaskStr = char(ssgateTask);

% Adjust finished states based on user task selection (never skips
% initialization)
if ~isempty(strfind(ssgateTaskStr,'Aim'))
    GpsFin = 1;
elseif ~isempty(strfind(ssgateTaskStr,'Start'))
    GpsFin = 1;
    AimFin = 1;
elseif ~isempty(strfind(ssgateTaskStr,'Speed'))
    GpsFin = 1;
    AimFin = 1;
end

% Set enable signals based on state completion
if GpsFin == 0
    GpsEn = 1;
    taskSelector = 1;
elseif AimFin == 0
    aimEn = 1;
    taskSelector = 2;
else
    deadEn = 1;
    taskSelector = 3;
end

== matlab function RobotX_ss_acoustics_1019_bbox/Main FSM/Acoustic FSM/Acoustics Pt3/Ping Point ==
  data: acousticPose output; Deployed input; Finished output; X input; Y input; Psi input; HorizBearing input; ElapsedTime input; Data output
function [acousticPose,Finished,Data] = PingPoint(Deployed,X,Y,Psi,...
    HorizBearing,ElapsedTime)
%Written by Anderson Lebbad on September 12, 2014
%Last Edited: September 14 - waits for boom deployment

%This function causes the vessel to spin in place until a ping is detected,
%then orients itself towards the direction of the source of that ping

persistent holdPose Pinged aveHeading First aveXY

if isempty(holdPose)
    holdPose = [X Y Psi];
    Pinged = 0;
    aveHeading = [0 0];
    aveXY = [0 0];
    First = 1;
end

%Initialize Data variable
Data = zeros(24,1);
Finished = 0;

%Angular offset (indirect rate control)
offset = 5;

%Wait for the boom to be lowered
if Deployed == 1
    %If the boat has not heard a ping yet, spin
    if Pinged == 0
        holdPose(3) = mod(Psi + offset,360);
    end
    
    %If the ping is less than 250 milliseconds (a timestep) then point at the
    %direction of sound
    if ElapsedTime < 250 && abs(HorizBearing) < 35
        if (abs(HorizBearing) >= 15 || First)
            holdPose(3) = mod(Psi + HorizBearing,360);
            Pinged = 1;
            First = 0;
        end
        aveHeading(1) = (aveHeading(1)*aveHeading(2)+Psi+HorizBearing)/(aveHeading(2)+1);
        aveHeading(2) = aveHeading(2)+1;
        aveXY(1) = (aveXY(1)*(aveHeading(2)-1)+X)/aveHeading(2);
        aveXY(2) = (aveXY(2)*(aveHeading(2)-1)+Y)/aveHeading(2);
    end
end

acousticPose = [aveXY aveHeading(1)];

if aveHeading(2) >= 16
    Finished = 1;
end

%Set desired pose
Data(1) = holdPose(1);
Data(2) = holdPose(2);
Data(3) = holdPose(3);

== matlab function RobotX_ss_acoustics_1019_bbox/Main FSM/Main Enabler ==
  data: taskSelector output; initEn output; startgateEn output; acouEn output; termEn output; RCEn output; OnOffRCAuto input; initFin input; startgateFin input; acouFin input
function [taskSelector,initEn,startgateEn,acouEn,termEn,RCEn] = taskEnabler(OnOffRCAuto,initFin,startgateFin,acouFin)
%Written by Anderson Lebbad on September 13, 2014
%Last Edited by:

%Changes the value of MainMode and the enablers for the tasks within the
%Main FSM.

% Initialize enable signals
RCEn = 0;
initEn = 0;
startgateEn = 0;
termEn = 0;
acouEn = 0;

% Set enable signals based on state completion
if initFin == 0
    initEn = 1;
    taskSelector = 1;
elseif OnOffRCAuto ~= 3
    RCEn = 1;
    taskSelector = 4;
elseif startgateFin == 0
    startgateEn = 1;
    taskSelector = 2;
elseif acouFin == 0
    acouEn = 1;
    taskSelector = 3;
else
    termEn = 1;
    taskSelector = 4;
end

== matlab function RobotX_ss_acoustics_1019_bbox/Main FSM/Acoustic FSM/Move 2/GPSMove ==
  data: GoalNED input; X input; Finished output; valid output; Y input; Psi input; pts output
function [Finished,valid,pts] = GPSmove(GoalNED,X,Y,Psi)
%Written by Dylan DeGaetano on September 1, 2014
%Last edited by: Anderson Lebbad
%
%This function will go to a given NED cooridnate, last edit changed the
%goal pt and variable names

persistent Sample
if isempty(Sample)
Sample = 0;
end
Finished = 0;
pts = zeros(8,2);
%$Distance to object in meters
if Sample == 100
    Sample = 0;
end

if Sample == 0
    pts(1,1) = X+5*cos(Psi*pi/180);
    pts(1,2) = Y+5*cos(Psi*pi/180);
    pts(8,1) = GoalNED(1,1);
    pts(8,2) = GoalNED(1,2);
    pts(2,:) = pts(1,:) +(1*(GoalNED-pts(1,:))/7);
    pts(3,:) = pts(1,:) +(2*(GoalNED-pts(1,:))/7);
    pts(4,:) = pts(1,:) +(3*(GoalNED-pts(1,:))/7);
    pts(5,:) = pts(1,:) +(4*(GoalNED-pts(1,:))/7);
    pts(6,:) = pts(1,:) +(5*(GoalNED-pts(1,:))/7);
    pts(7,:) = pts(1,:) +(6*(GoalNED-pts(1,:))/7);
    Sample = 1; 
    valid = 1;
    
else 
    range = sqrt(sum((GoalNED - [X Y]).^2));
    if range <= 5
        Finished = 1;
    end
    valid = 0;
    Sample = Sample + 1;
end

== matlab function RobotX_ss_acoustics_1019_bbox/Main FSM/Acoustic FSM/Move 3/CalcTimes ==
  data: pts input; u input; Data output
function Data = calcTimes(pts, u)
%Written by Anderson Lebbad on August 9, 2014
%Last Edited: Dylan DeGaetano September 1, 2014

%Calculates times for the boat to get to points for a trajectory, and
%formats Data for communication

%Initialize
Data = zeros(24,1);
traj = zeros(8,3);
traj(:,1:2) = pts;



for k = 2:8
    %Calculate distance to travel from last point
    distTravel = sqrt(sum((pts(k-1,:)-pts(k,:)).^2));
    %Assume 1m per second speed
    traj(k,3) = traj(k-1,3) + distTravel;
    %Add time based off initial velocity to get to first point past initial
    if k == 2
        traj(k,3) = traj(k,3) + 2.5*abs(2-u);
    end
end


%Output Data
for i=1:8
    for j = 1:3
        Data(3*(i-1)+j) = traj(i,j);
    end
end

== matlab function RobotX_ss_acoustics_1019_bbox/Main FSM/Acoustic FSM/Move 3/GPSMove ==
  data: GoalNED input; X input; Finished output; valid output; Y input; Psi input; pts output
function [Finished,valid,pts] = GPSmove(GoalNED,X,Y,Psi)
%Written by Dylan DeGaetano on September 1, 2014
%Last edited by: Anderson Lebbad
%
%This function will go to a given NED cooridnate, last edit changed the
%goal pt and variable names

persistent Sample
if isempty(Sample)
Sample = 0;
end
Finished = 0;
pts = zeros(8,2);
%$Distance to object in meters
if Sample == 100
    Sample = 0;
end

if Sample == 0
    pts(1,1) = X+5*cos(Psi*pi/180);
    pts(1,2) = Y+5*cos(Psi*pi/180);
    pts(8,1) = GoalNED(1,1);
    pts(8,2) = GoalNED(1,2);
    pts(2,:) = pts(1,:) +(1*(GoalNED-pts(1,:))/7);
    pts(3,:) = pts(1,:) +(2*(GoalNED-pts(1,:))/7);
    pts(4,:) = pts(1,:) +(3*(GoalNED-pts(1,:))/7);
    pts(5,:) = pts(1,:) +(4*(GoalNED-pts(1,:))/7);
    pts(6,:) = pts(1,:) +(5*(GoalNED-pts(1,:))/7);
    pts(7,:) = pts(1,:) +(6*(GoalNED-pts(1,:))/7);
    Sample = 1; 
    valid = 1;
    
else 
    range = sqrt(sum((GoalNED - [X Y]).^2));
    if range <= 5
        Finished = 1;
    end
    valid = 0;
    Sample = Sample + 1;
end

== matlab function RobotX_ss_acoustics_1019_bbox/Main FSM/Start//Speedgate/GPS Move/LLA to NED ==
  data: GoalLLA input; GoalNED output; NED_origin input
function GoalNED = LLA2NEDfun(GoalLLA,NED_origin)
%Written by Anderson Lebbad on September 20, 2014
%Last edited by:
%
%This function converts a target Latitude, Longitude, Altitude (LLA) point
%into North, East, Down (NED) coordinates

%First convert to earth centered, earth fixed frame
GoalECEF = lla2ecef([GoalLLA*(pi/180), 0]');
%Then convert from ECEF to North East Down
GoalNEDvect = ecef2ned(NED_origin'*(pi/180),GoalECEF);
GoalNED = GoalNEDvect(1:2)';

end

function x_ecef = lla2ecef(x_lla)
% LLE2ECEF: Converts from geodetic latitude, longitude, and altitude to earth-centered earth-fixed Cartesian coordinates
% INPUT: latitude phi (rad), longitude lambda (rad), altitude h (m)
% OUTPUT: [x, y, z]' (m) earth-centered earth-fixed Cartesian coordinates
    a = 6378137; % equatorial radius of ellipsoid (semi-major axis) (m)
    b = 6356752; % polar axis radius of ellipsoid (semi-minor axis) (m)

    phi = x_lla(1);
    lambda = x_lla(2);
    h = x_lla(3);
    
    % auxiliar quantities f, e, and N
    f = (a-b)/a;
    e = f*(2-f);
    N = a/sqrt(1-(e*sin(phi))^2);
    x_ecef = [(N+h)*cos(phi)*cos(lambda); (N+h)*cos(phi)*sin(lambda); (N*(1-e^2)+h)*sin(phi)];
end

function [x_ned] = ecef2ned(ned_lla, x_ecef)
% ECEF2NED Converts from earth-centered, earth-fixed Cartesian coordinates to tangent plane
% INPUT:
% 1) x_ecef=[x,y,z]' (m) earth-centered, earth-fixed Cartesian coordinates
% 2) ned_lla=[phi,lambda]' consiting of latitude phi (rad), longitude lambda (rad) of NED origin
% OUTPUT:
% 1) x_ned=[x,y,z]' (m) in NED coordinate system with the origin [phi,lambda]'

    phi = ned_lla(1);
    lambda = ned_lla(2);

    % transformation  matrix
    T = [-sin(phi)*cos(lambda) -sin(phi)*sin(lambda)  cos(phi)
         -sin(lambda)           cos(lambda)           0
          cos(phi)*cos(lambda)   cos(phi)*sin(lambda)  sin(phi)];

     x_ned = T*(x_ecef-lla2ecef([phi, lambda, 0]')); % convert to NED
     x_ned(3) = -x_ned(3);
end

== matlab function RobotX_ss_acoustics_1019_bbox/Sensors/Serial In/MATLAB Function ==
  data: Time input; asciiHRT output; Lat input; Long input; Mode input; Task input
% This function creates the heartbeat message to be sent from Speedgoat in
% ascii code
% Written by: Edward Zhu
% Date: 9/17/14

function asciiHRT = asciiHRTEncoder(Time, Lat, Long, Mode, Task)

% Initialize output message vector as the serial output block expects 128
% character message
asciiHRT = uint8(zeros(1,128));

% Convert static strings to ascii code
asciiMsgID = uint8('$RXHRT,');
asciiComma = uint8(',');
asciiDeciPt = uint8('.');
if Lat >= 0
    asciiNS = uint8('N,');
else
    Lat = -Lat;
    asciiNS = uint8('S,');
end
if Long >= 0
    asciiEW = uint8('E,');
else
    Long = -Long;
    asciiEW = uint8('W,');
end
asciiTeamID = uint8('AUVSI,');
asciiMsgEnd = uint8('*');
asciiMsgCRLF = [13 10];

% Convert UTC Time input (hhmmss) into ascii code
asciiTime = uint8(zeros(1,7));
asciiTime(7) = asciiComma;

for timeChar = 1:6
    asciiTime(timeChar) = floor(mod(Time,10^(7-timeChar))/...
        10^(6-timeChar)) + 48;
end

% Convert latitude (dd.mmmmmm) into ascii code
asciiLat = uint8(zeros(1,10));
asciiLat(10) = asciiComma;
asciiLat(3) = asciiDeciPt;

latInt = floor(Lat);
for latIntChar = 1:2
    asciiLat(latIntChar) = floor(mod(latInt,10^(3-latIntChar))/...
        10^(2-latIntChar)) + 48;
end

latDeci = mod(Lat,latInt) * 10^6;
for latDeciChar = 1:6
    asciiLat(latDeciChar+3) = floor(mod(latDeci,10^(7-latDeciChar))/...
        10^(6-latDeciChar)) + 48;
end

% Convert longitude (ddd.mmmmmm) into ascii code
asciiLong = uint8(zeros(1,11));
asciiLong(11) = asciiComma;
asciiLong(4) = asciiDeciPt;

longInt = floor(Long);
for longIntChar = 1:3
    asciiLong(longIntChar) = floor(mod(longInt,10^(4-longIntChar))/...
        10^(3-longIntChar)) + 48;
end

longDeci = mod(Long,longInt) * 10^6;
for longDeciChar = 1:6
    asciiLong(longDeciChar+4) = floor(mod(longDeci,10^(7-longDeciChar))/...
        10^(6-longDeciChar)) + 48;
end

% Convert vehicle mode into ascii (1 = RC, 2 = Auto)
asciiMode = [uint8(Mode+48) asciiComma];

% Convert vehicle task into ascii
asciiTask = [uint8(Task+48) asciiMsgEnd];

% Concat individual ascii arrays into one array
asciiPreChkSum = cat(2,asciiMsgID,asciiTime,asciiLat,asciiNS,asciiLong,asciiEW,...
    asciiTeamID,asciiMode,asciiTask);

% Calculate the checksum of the message from the '$' to the '*' and convert
% to hex
chkSum = uint8(0);

for chksumChar = 1:(length(asciiPreChkSum)-2)
    chkSum = bitxor(chkSum,asciiPreChkSum(chksumChar+1));
end

% Convert the checksum to ascii
chkSum = dec2hex(chkSum);
asciiChkSum = uint8(zeros(1,length(chkSum))+32);
for i = 1:length(chkSum)
    asciiChkSum(i) = uint8(chkSum(i));
end

% Concat the checksum and the '/r/n' to the end of the message
asciiPostChkSum = cat(2,asciiPreChkSum,asciiChkSum,asciiMsgCRLF);

% Output the final message
asciiHRT(1:length(asciiPostChkSum)) = asciiPostChkSum;

== matlab function RobotX_ss_acoustics_1019_bbox/Sensors/Serial In/Data Update1 ==
  data: Valid input; ControlMode input; V output; C output; L output; A output; Data input; D1 output; D2 output; D3 output; D4 output; D5 output; D6 output; D7 output; D8 output; D9 output; D10 output; D11 output; D12 output; D13 output; D14 output; D15 output; D16 output; D17 output; D18 output; D19 output; D20 output; D21 output; D22 output; D23 output; D24 output; Activate input
function [V,C,L,A,D1,D2,D3,D4,D5,D6,D7,D8,D9,D10,D11,D12,D13,D14,D15,D16,D17,...
    D18,D19,D20,D21,D22,D23,D24] = dataSplit(Valid,ControlMode,Data,Activate)
%Written by Anderson Lebbad on August 10, 2014
%Last Edited by: Anderson Lebbad on September 11, 2014

%This function splits the data vector into the twelve channels it is
%composed of for communication

persistent HoldData

A = Activate;

if isempty(HoldData)
    HoldData = zeros(26,1);
end

L = 8;

if Valid == 1
    HoldData(1) = Valid;
    HoldData(2) = ControlMode;
    HoldData(3) = Data(1);
    HoldData(4) = Data(2);
    HoldData(5) = Data(3);
    HoldData(6) = Data(4);
    HoldData(7) = Data(5);
    HoldData(8) = Data(6);
    HoldData(9) = Data(7);
    HoldData(10) = Data(8);
    HoldData(11) = Data(9);
    HoldData(12) = Data(10);
    HoldData(13) = Data(11);
    HoldData(14) = Data(12);
    HoldData(15) = Data(13);
    HoldData(16) = Data(14);
    HoldData(17) = Data(15);
    HoldData(18) = Data(16);
    HoldData(19) = Data(17);
    HoldData(20) = Data(18);
    HoldData(21) = Data(19);
    HoldData(22) = Data(20);
    HoldData(23) = Data(21);
    HoldData(24) = Data(22);
    HoldData(25) = Data(23);
    HoldData(26) = Data(24);
end

V = HoldData(1);
C = HoldData(2);
D1 = HoldData(3);
D2 = HoldData(4);
D3 = HoldData(5);
D4 = HoldData(6);
D5 = HoldData(7);
D6 = HoldData(8);
D7 = HoldData(9);
D8 = HoldData(10);
D9 = HoldData(11);
D10 = HoldData(12);
D11 = HoldData(13);
D12 = HoldData(14);
D13 = HoldData(15);
D14 = HoldData(16);
D15 = HoldData(17);
D16 = HoldData(18);
D17 = HoldData(19);
D18 = HoldData(20);
D19 = HoldData(21);
D20 = HoldData(22);
D21 = HoldData(23);
D22 = HoldData(24);
D23 = HoldData(25);
D24 = HoldData(26);

end
